simulink model "simulaciones0ct28"  (R2013b)
settings: Solver=ode45  StartTime=0.0  StopTime=0.3  RelTol=1e-3
libraries: powerlib x31
settings Model: Creator=ricardo  LastModifiedBy=Ricardo
settings DataIOCC: SignalLoggingSaveFormat=ModelDataLogs
settings DebuggingCC: UnderspecifiedInitializationDetection=Simplified  MultiTaskDSMMsg=warning  MultiTaskCondExecSysMsg=none
settings RTWCC: IncludeERTFirstTime=on
settings GRTTargetCC: CodeReplacementLibrary=None  CPPClassGenCompliant=on

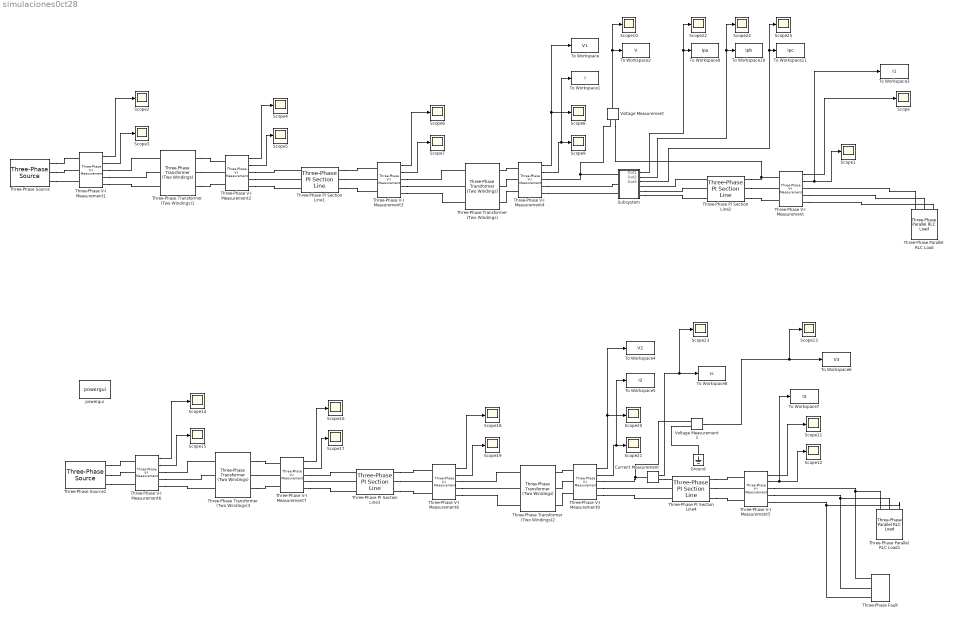
== system simulaciones0ct28 ==
  Current Measurement : powerlib/Measurements/Current Measurement  PhasorSimulation=off  OutputType=Complex  PSBequivalent=0
  Ground : powerlib/Elements/Ground  LConnTagsString=a
  Scope{,1..25} (26 alike) : Scope
      Scope settings: YMin=-20000  YMax=20000
      Scope1 settings: YMin=-3000  YMax=3500
      Scope10 settings: YMin=-20000  YMax=20000  SaveName=ScopeData10
      Scope11 settings: YMin=-20000  YMax=20000  SaveName=ScopeData11
      Scope12 settings: YMin=-3000  YMax=3500  SaveName=ScopeData12
      Scope13 settings: YMin=-20000  YMax=20000  SaveName=ScopeData13
      Scope14 settings: YMin=-175000  YMax=175000  SaveName=ScopeData14
      Scope15 settings: YMin=-700  YMax=700  SaveName=ScopeData15
      Scope16 settings: YMin=-20000  YMax=20000  SaveName=ScopeData16
      Scope17 settings: YMin=-20000  YMax=20000  SaveName=ScopeData17
      Scope18 settings: YMin=-20000  YMax=20000  SaveName=ScopeData18
      Scope19 settings: YMin=-900  YMax=900  SaveName=ScopeData19
      Scope2 settings: YMin=-175000  YMax=175000  SaveName=ScopeData2
      Scope20 settings: YMin=-20000  YMax=20000  SaveName=ScopeData20
      Scope21 settings: YMin=-20000  YMax=20000  SaveName=ScopeData21
      Scope22 settings: YMin=-20000  YMax=20000  SaveName=ScopeData22
      Scope23 settings: YMin=-20000  YMax=20000  SaveName=ScopeData23
      Scope24 settings: YMin=-20000  YMax=20000  SaveName=ScopeData24
      Scope25 settings: YMin=-20000  YMax=20000  SaveName=ScopeData25
      Scope3 settings: YMin=-700  YMax=700  SaveName=ScopeData3
      Scope4 settings: YMin=-20000  YMax=20000  SaveName=ScopeData4
      Scope5 settings: YMin=-20000  YMax=20000  SaveName=ScopeData5
      Scope6 settings: YMin=-20000  YMax=20000  SaveName=ScopeData6
      Scope7 settings: YMin=-900  YMax=900  SaveName=ScopeData7
      Scope8 settings: YMin=-20000  YMax=20000  SaveName=ScopeData8
      Scope9 settings: YMin=-20000  YMax=20000  SaveName=ScopeData9
  Subsystem : Subsystem
  Three-Phase PI Section Line1 : powerlib/Elements/Three-Phase PI Section Line  LConnTagsString=a|b|c  RConnTagsString=A|B|C  Frequency=60  Resistances=[ 0.41586 0.82784]  Inductances="[ 1.3743e-3  4.2583e-3]"  Capacitances=[0.00825e-6 0.00588e-6]  Length=9
  Three-Phase PI Section Line2 : powerlib/Elements/Three-Phase PI Section Line  LConnTagsString=a|b|c  RConnTagsString=A|B|C  Frequency=60  Resistances=[ 0.41586 0.82784]  Inductances="[ 1.3743e-3  4.2583e-3]"  Capacitances=[0.00825e-6 0.00588e-6]  Length=3
  Three-Phase PI Section Line3 : powerlib/Elements/Three-Phase PI Section Line  LConnTagsString=a|b|c  RConnTagsString=A|B|C  Frequency=60  Resistances=[ 0.41586 0.82784]  Inductances="[ 1.3743e-3  4.2583e-3]"  Capacitances=[0.00825e-6 0.00588e-6]  Length=10
  Three-Phase PI Section Line4 : powerlib/Elements/Three-Phase PI Section Line  LConnTagsString=a|b|c  RConnTagsString=A|B|C  Frequency=60  Resistances=[ 0.41586 0.82784]  Inductances="[ 1.3743e-3  4.2583e-3]"  Capacitances=[0.00825e-6 0.00588e-6]  Length=0.26386
  Three-Phase Parallel RLC Load : powerlib/Elements/Three-Phase Parallel RLC Load  LConnTagsString=A|B|C  Configuration=Y (grounded)  NominalVoltage=13800  NominalFrequency=60  ActivePower=13800  InductivePower=0  CapacitivePower=0  Measurements=None  LoadType=constant Z
  Three-Phase Parallel RLC Load1 : powerlib/Elements/Three-Phase Parallel RLC Load  LConnTagsString=A|B|C  Configuration=Y (grounded)  NominalVoltage=13800  NominalFrequency=60  ActivePower=13800  InductivePower=0  CapacitivePower=0  Measurements=None  LoadType=constant Z
  Three-Phase Transformer (Two Windings) : powerlib/Elements/Three-Phase Transformer (Two Windings)  Winding1Connection=Yg  UNITS=pu  NominalPower=[ 5e6 , 60 ]  Winding1=[ 34500 , 0 , 0.0273 ]  Winding2Connection=Yg  Winding2=[ 13800 , 0 , 0.0273 ]  SetSaturation=off  Rm=500  Lm=500  Saturation=[ 0,0 ; 0.0024,1.2 ; 1.0,1.52 ]  Hysteresis=off  DataFile='hysteresis'  SetInitialFlux=off  InitialFluxes=[ 0.8 , -0.8 , 0.7 ]  Measurements=None  MoreParameters=off  BreakLoop=off  DataType=off  TransfoNumber=1
  Three-Phase Transformer (Two Windings)1 : powerlib/Elements/Three-Phase Transformer (Two Windings)  Winding1Connection=Yg  UNITS=pu  NominalPower=[ 40e6 , 60 ]  Winding1=[ 115000 , 0 , 0.06 ]  Winding2Connection=Yg  Winding2=[ 34500 , 0 , 0.06 ]  SetSaturation=off  Rm=500  Lm=500  Saturation=[ 0,0 ; 0.0024,1.2 ; 1.0,1.52 ]  Hysteresis=off  DataFile='hysteresis'  SetInitialFlux=off  InitialFluxes=[ 0.8 , -0.8 , 0.7 ]  Measurements=None  MoreParameters=off  BreakLoop=off  DataType=off  TransfoNumber=1
  Three-Phase Transformer (Two Windings)2 : powerlib/Elements/Three-Phase Transformer (Two Windings)  Winding1Connection=Yg  UNITS=pu  NominalPower=[ 5e6 , 60 ]  Winding1=[ 34500 , 0 , 0.0273 ]  Winding2Connection=Yg  Winding2=[ 13800 , 0 , 0.0273 ]  SetSaturation=off  Rm=500  Lm=500  Saturation=[ 0,0 ; 0.0024,1.2 ; 1.0,1.52 ]  Hysteresis=off  DataFile='hysteresis'  SetInitialFlux=off  InitialFluxes=[ 0.8 , -0.8 , 0.7 ]  Measurements=None  MoreParameters=off  BreakLoop=off  DataType=off  TransfoNumber=1
  Three-Phase Transformer (Two Windings)3 : powerlib/Elements/Three-Phase Transformer (Two Windings)  Winding1Connection=Yg  UNITS=pu  NominalPower=[ 40e6 , 60 ]  Winding1=[ 115000 , 0 , 0.06 ]  Winding2Connection=Yg  Winding2=[ 34500 , 0 , 0.06 ]  SetSaturation=off  Rm=500  Lm=500  Saturation=[ 0,0 ; 0.0024,1.2 ; 1.0,1.52 ]  Hysteresis=off  DataFile='hysteresis'  SetInitialFlux=off  InitialFluxes=[ 0.8 , -0.8 , 0.7 ]  Measurements=None  MoreParameters=off  BreakLoop=off  DataType=off  TransfoNumber=1
  Three-Phase V-I Measurement{,4..5,9} (4 alike) : powerlib/Measurements/Three-Phase V-I Measurement  VoltageMeasurement=phase-to-ground  SetLabelV=off  LabelV=Vabc  Vpu=off  VpuLL=off  CurrentMeasurement=yes  SetLabelI=off  LabelI=Iabc  Ipu=off  Pbase=100e6  Vbase=500e3  OutputType=Complex  PhasorSimulation=off  PSBequivalent=0
  Three-Phase V-I Measurement{1..3,6..8} (6 alike) : powerlib/Measurements/Three-Phase V-I Measurement  VoltageMeasurement=phase-to-phase  SetLabelV=off  LabelV=Vabc  Vpu=off  VpuLL=off  CurrentMeasurement=yes  SetLabelI=off  LabelI=Iabc  Ipu=off  Pbase=100e6  Vbase=500e3  OutputType=Complex  PhasorSimulation=off  PSBequivalent=0
  Three-Phase Fault : powerlib/Elements/Three-Phase Fault  FaultA=on  FaultB=off  FaultC=off  FaultResistance=0.001  GroundFault=on  GroundResistance=6.94  External=off  SwitchStatus=[1 0]  SwitchTimes="[0.05  0.15]"  InitialStates=[0 0 1]  SnubberResistance=1e6  SnubberCapacitance=inf  Measurements=Fault currents
  Three-Phase Source : powerlib/Electrical Sources/Three-Phase Source  Voltage=115000  PhaseAngle=120  Frequency=60  InternalConnection=Yg  SpecifyImpedance=on  Resistance=0.8929  Inductance=16.58e-3  ShortCircuitLevel=100e6  BaseVoltage=115000  XRratio=7  BusType=swing  Pref=0  Qref=0  Qmin=-inf  Qmax=inf
  Three-Phase Source1 : powerlib/Electrical Sources/Three-Phase Source  Voltage=115000  PhaseAngle=120  Frequency=60  InternalConnection=Yg  SpecifyImpedance=on  Resistance=0.8929  Inductance=16.58e-3  ShortCircuitLevel=100e6  BaseVoltage=115000  XRratio=7  BusType=swing  Pref=0  Qref=0  Qmin=-inf  Qmax=inf
  To Workspace : ToWorkspace  VariableName=V1  SampleTime=-1
  To Workspace1 : ToWorkspace  VariableName=I  SampleTime=-1
  To Workspace10 : ToWorkspace  VariableName=Ipb  SampleTime=-1
  To Workspace11 : ToWorkspace  VariableName=Ipc  SampleTime=-1
  To Workspace2 : ToWorkspace  VariableName=V  SampleTime=-1
  To Workspace3 : ToWorkspace  VariableName=I1  SampleTime=-1
  To Workspace4 : ToWorkspace  VariableName=V2  SampleTime=-1
  To Workspace5 : ToWorkspace  VariableName=I2  SampleTime=-1
  To Workspace6 : ToWorkspace  VariableName=V3  SampleTime=-1
  To Workspace7 : ToWorkspace  VariableName=I3  SampleTime=-1  SaveFormat=Structure With Time
  To Workspace8 : ToWorkspace  VariableName=Is  SampleTime=-1
  To Workspace9 : ToWorkspace  VariableName=Ipa  SampleTime=-1
  Voltage Measurement : powerlib/Measurements/Voltage Measurement  PhasorSimulation=off  OutputType=Complex  PSBequivalent=0
  Voltage Measurement1 : powerlib/Measurements/Voltage Measurement  PhasorSimulation=off  OutputType=Complex  PSBequivalent=0
  powergui : powerlib/powergui  Priority=1  SimulationMode=Discrete  SolverType=Tustin  SampleTime=5.208333e-4  frequency=60  SPID=off  DisableSnubberDevices=off  DisableRonSwitches=off  DisableVfSwitches=off  SwTol=0  Interpol=off  DisplayEquations=off  frequencyindice=60  Pbase=100e6  ErrMax=1e-4  Iterations=50  UnitsV=kV  UnitsW=MW  FunctionMessages=off  echomessages=off  HookPort=off  EnableUseOfTLC=off  x0status=blocks  RestoreLinks=warning  ResistiveCurrentMeasurement=off  Frange=[0:2:500]  Ylog=off  Xlog=on  ShowGrid=off  save=off  variable=ZData  structure=0  ZoomFFT=off  StartTime=0.0  cycles=1  DisplayStyle=1  fundamental=60  FreqAxis=off  MaxFrequency=1000  frequencyindicesteady=1  RmsSteady=1  display=off  Ts=0  methode=off
  wires:
  Three-Phase V-I Measurement/1 -> Scope/1
  Three-Phase V-I Measurement/2 -> To Workspace3/1, Scope1/1
  Three-Phase V-I Measurement1/1 -> Scope2/1
  Three-Phase V-I Measurement1/2 -> Scope3/1
  Three-Phase V-I Measurement2/1 -> Scope4/1
  Three-Phase V-I Measurement2/2 -> Scope5/1
  Three-Phase V-I Measurement3/1 -> Scope6/1
  Three-Phase V-I Measurement3/2 -> Scope7/1
  Three-Phase V-I Measurement4/1 -> Scope8/1, To Workspace/1
  Three-Phase V-I Measurement4/2 -> To Workspace1/1, Scope9/1
  Voltage Measurement/1 -> To Workspace2/1, Scope10/1
  Three-Phase V-I Measurement5/1 -> Scope11/1
  Three-Phase V-I Measurement5/2 -> To Workspace7/1, Scope12/1
  Three-Phase V-I Measurement6/1 -> Scope14/1
  Three-Phase V-I Measurement6/2 -> Scope15/1
  Three-Phase V-I Measurement7/1 -> Scope16/1
  Three-Phase V-I Measurement7/2 -> Scope17/1
  Three-Phase V-I Measurement8/1 -> Scope18/1
  Three-Phase V-I Measurement8/2 -> Scope19/1
  Three-Phase V-I Measurement9/1 -> Scope20/1, To Workspace4/1
  Three-Phase V-I Measurement9/2 -> To Workspace5/1, Scope21/1
  Voltage Measurement1/1 -> Scope13/1, To Workspace6/1
  Current Measurement/1 -> Scope23/1, To Workspace8/1
  Subsystem/1(Out1) -> To Workspace9/1, Scope22/1
  Subsystem/2(Out2) -> To Workspace10/1, Scope24/1
  Subsystem/3(Out3) -> To Workspace11/1, Scope25/1
  connections:
  Three-Phase PI Section Line2/RConn1 -- Voltage Measurement/LConn2 -- Three-Phase V-I Measurement/LConn1
  Three-Phase PI Section Line2/RConn2 -- Three-Phase V-I Measurement/LConn2
  Three-Phase PI Section Line2/RConn3 -- Three-Phase V-I Measurement/LConn3
  Three-Phase V-I Measurement/RConn1 -- Three-Phase Parallel RLC Load/LConn1
  Three-Phase V-I Measurement/RConn2 -- Three-Phase Parallel RLC Load/LConn2
  Three-Phase V-I Measurement/RConn3 -- Three-Phase Parallel RLC Load/LConn3
  Three-Phase Source/RConn1 -- Three-Phase V-I Measurement1/LConn1
  Three-Phase Source/RConn2 -- Three-Phase V-I Measurement1/LConn2
  Three-Phase Source/RConn3 -- Three-Phase V-I Measurement1/LConn3
  Three-Phase V-I Measurement1/RConn1 -- Three-Phase Transformer (Two Windings)1/LConn1
  Three-Phase V-I Measurement1/RConn2 -- Three-Phase Transformer (Two Windings)1/LConn2
  Three-Phase V-I Measurement1/RConn3 -- Three-Phase Transformer (Two Windings)1/LConn3
  Three-Phase Transformer (Two Windings)1/RConn1 -- Three-Phase V-I Measurement2/LConn1
  Three-Phase Transformer (Two Windings)1/RConn2 -- Three-Phase V-I Measurement2/LConn2
  Three-Phase Transformer (Two Windings)1/RConn3 -- Three-Phase V-I Measurement2/LConn3
  Three-Phase V-I Measurement2/RConn1 -- Three-Phase PI Section Line1/LConn1
  Three-Phase V-I Measurement2/RConn2 -- Three-Phase PI Section Line1/LConn2
  Three-Phase V-I Measurement2/RConn3 -- Three-Phase PI Section Line1/LConn3
  Three-Phase PI Section Line1/RConn1 -- Three-Phase V-I Measurement3/LConn1
  Three-Phase PI Section Line1/RConn2 -- Three-Phase V-I Measurement3/LConn2
  Three-Phase PI Section Line1/RConn3 -- Three-Phase V-I Measurement3/LConn3
  Three-Phase V-I Measurement3/RConn2 -- Three-Phase Transformer (Two Windings)/LConn2
  Three-Phase V-I Measurement3/RConn3 -- Three-Phase Transformer (Two Windings)/LConn3
  Three-Phase V-I Measurement3/RConn1 -- Three-Phase Transformer (Two Windings)/LConn1
  Three-Phase Transformer (Two Windings)/RConn1 -- Three-Phase V-I Measurement4/LConn1
  Three-Phase Transformer (Two Windings)/RConn2 -- Three-Phase V-I Measurement4/LConn2
  Three-Phase Transformer (Two Windings)/RConn3 -- Three-Phase V-I Measurement4/LConn3
  Three-Phase V-I Measurement4/RConn1 -- Subsystem/LConn1 -- Voltage Measurement/LConn1
  Three-Phase V-I Measurement4/RConn2 -- Subsystem/LConn2
  Three-Phase V-I Measurement4/RConn3 -- Subsystem/LConn3
  Three-Phase PI Section Line4/RConn1 -- Three-Phase V-I Measurement5/LConn1
  Three-Phase Parallel RLC Load1/LConn1 -- Three-Phase Fault/LConn1 -- Three-Phase V-I Measurement5/RConn1
  Three-Phase Parallel RLC Load1/LConn2 -- Three-Phase Fault/LConn2 -- Three-Phase V-I Measurement5/RConn2
  Three-Phase Parallel RLC Load1/LConn3 -- Three-Phase Fault/LConn3 -- Three-Phase V-I Measurement5/RConn3
  Three-Phase V-I Measurement9/RConn1 -- Current Measurement/LConn1 -- Voltage Measurement1/LConn1
  Three-Phase Transformer (Two Windings)2/RConn2 -- Three-Phase V-I Measurement9/LConn2
  Three-Phase V-I Measurement8/RConn2 -- Three-Phase Transformer (Two Windings)2/LConn2
  Three-Phase Transformer (Two Windings)3/RConn1 -- Three-Phase V-I Measurement7/LConn1
  Three-Phase V-I Measurement9/RConn2 -- Three-Phase PI Section Line4/LConn2
  Three-Phase V-I Measurement6/RConn2 -- Three-Phase Transformer (Two Windings)3/LConn2
  Three-Phase PI Section Line4/RConn3 -- Three-Phase V-I Measurement5/LConn3
  Three-Phase Source1/RConn2 -- Three-Phase V-I Measurement6/LConn2
  Three-Phase V-I Measurement7/RConn3 -- Three-Phase PI Section Line3/LConn3
  Three-Phase PI Section Line4/RConn2 -- Three-Phase V-I Measurement5/LConn2
  Three-Phase Transformer (Two Windings)2/RConn3 -- Three-Phase V-I Measurement9/LConn3
  Three-Phase V-I Measurement6/RConn3 -- Three-Phase Transformer (Two Windings)3/LConn3
  Three-Phase Transformer (Two Windings)3/RConn3 -- Three-Phase V-I Measurement7/LConn3
  Three-Phase Source1/RConn3 -- Three-Phase V-I Measurement6/LConn3
  Three-Phase PI Section Line3/RConn1 -- Three-Phase V-I Measurement8/LConn1
  Three-Phase V-I Measurement6/RConn1 -- Three-Phase Transformer (Two Windings)3/LConn1
  Three-Phase PI Section Line3/RConn3 -- Three-Phase V-I Measurement8/LConn3
  Three-Phase V-I Measurement8/RConn1 -- Three-Phase Transformer (Two Windings)2/LConn1
  Three-Phase V-I Measurement8/RConn3 -- Three-Phase Transformer (Two Windings)2/LConn3
  Three-Phase V-I Measurement7/RConn2 -- Three-Phase PI Section Line3/LConn2
  Three-Phase PI Section Line3/RConn2 -- Three-Phase V-I Measurement8/LConn2
  Three-Phase Transformer (Two Windings)2/RConn1 -- Three-Phase V-I Measurement9/LConn1
  Three-Phase V-I Measurement9/RConn3 -- Three-Phase PI Section Line4/LConn3
  Three-Phase V-I Measurement7/RConn1 -- Three-Phase PI Section Line3/LConn1
  Three-Phase Source1/RConn1 -- Three-Phase V-I Measurement6/LConn1
  Three-Phase Transformer (Two Windings)3/RConn2 -- Three-Phase V-I Measurement7/LConn2
  Current Measurement/RConn1 -- Three-Phase PI Section Line4/LConn1
  Ground/LConn1 -- Voltage Measurement1/LConn2
  Three-Phase PI Section Line2/LConn1 -- Subsystem/RConn1
  Subsystem/RConn2 -- Three-Phase PI Section Line2/LConn2
  Subsystem/RConn3 -- Three-Phase PI Section Line2/LConn3

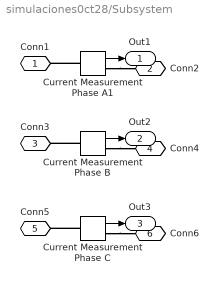
== system simulaciones0ct28/Subsystem ==
  Current Measurement Phase A1 : powerlib/Measurements/Current Measurement  PhasorSimulation=off  OutputType=Complex  PSBequivalent=0
  Current Measurement Phase B : powerlib/Measurements/Current Measurement  PhasorSimulation=off  OutputType=Complex  PSBequivalent=0
  Current Measurement Phase C : powerlib/Measurements/Current Measurement  PhasorSimulation=off  OutputType=Complex  PSBequivalent=0
  Conn1 : PMIOPort  Port=1  Side=Left
  Conn2 : PMIOPort  Port=2  Side=Right
  Conn3 : PMIOPort  Port=3  Side=Left
  Conn4 : PMIOPort  Port=4  Side=Right
  Conn5 : PMIOPort  Port=5  Side=Left
  Conn6 : PMIOPort  Port=6  Side=Right
  Out1 : Outport
  Out2 : Outport  Port=2
  Out3 : Outport  Port=3
  wires:
  Current Measurement Phase A1/1 -> Out1/1
  Current Measurement Phase B/1 -> Out2/1
  Current Measurement Phase C/1 -> Out3/1
  connections:
  Current Measurement Phase A1/LConn1 -- Conn1/RConn1
  Current Measurement Phase C/RConn1 -- Conn6/RConn1
  Current Measurement Phase C/LConn1 -- Conn5/RConn1
  Current Measurement Phase A1/RConn1 -- Conn2/RConn1
  Current Measurement Phase B/LConn1 -- Conn3/RConn1
  Current Measurement Phase B/RConn1 -- Conn4/RConn1
